simulink model "Copy_of_Esercizio8_sim"  (R2022a)
settings: Solver=VariableStepAuto  StartTime=0.0  StopTime=60  RelTol=1e-3
values from neighbouring files (symbols this model uses):
  PID_d = c2d (PID_continuo, Ts,'tustin')    [PID.m]
  Ts = 1/100    (= 0.01)    [PID.m]
undefined symbols (not defined in the file or in its folder): PI_discreto, PID_discreto
settings Model: Creator=chiar  LastModifiedBy=Stefano
settings SolverCC: AlgebraicLoopSolver=TrustRegion
settings DebuggingCC: UnconnectedInputMsg=warning  UnconnectedOutputMsg=warning  UnconnectedLineMsg=warning  SFMachineParentedDataDiag=warning
settings RTWCC: DLArmComputeVersion=19.05

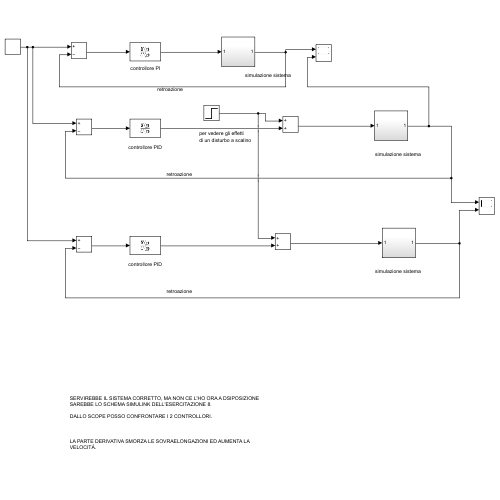
[thumbnail: Simulink's stored preview of the top-level diagram]
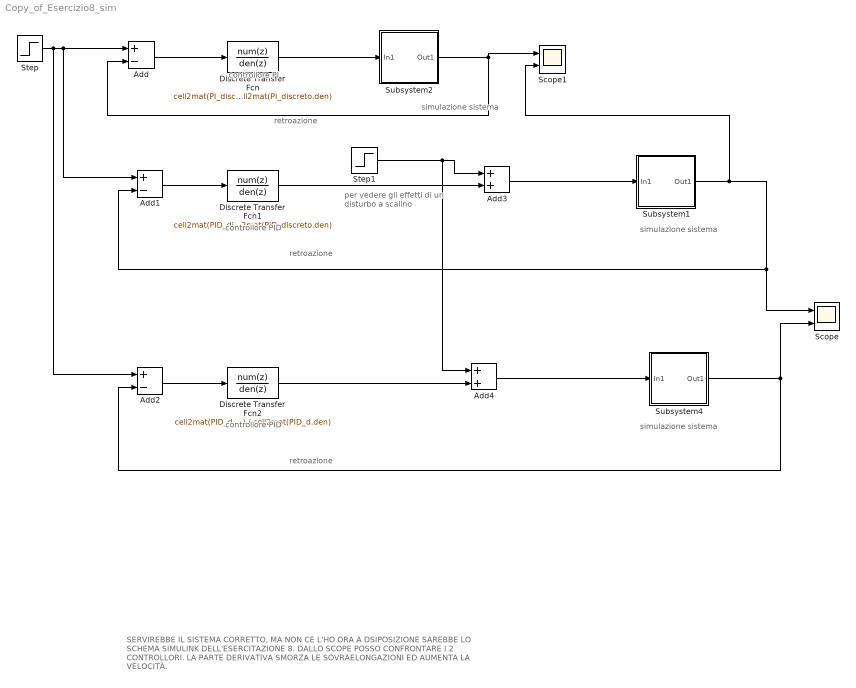
== system Copy_of_Esercizio8_sim ==
  note: per vedere gli effetti
      | di un disturbo a scalino
  note: SERVIREBBE IL SISTEMA CORRETTO, MA NON CE L'HO ORA A DSIPOSIZIONE
      | SAREBBE LO SCHEMA SIMULINK DELL'ESERCITAZIONE 8.
      |
      | DALLO SCOPE POSSO CONFRONTARE I 2 CONTROLLORI.
      |
      |
      |
      | LA PARTE DERIVATIVA SMORZA LE SOVRAELONGAZIONI ED AUMENTA LA VELOCITÀ.
  note: retroazione
  note: simulazione sistema
  note: controllore PID
  note: controllore PI
  note: simulazione sistema
  note: retroazione
  note: simulazione sistema
  note: controllore PID
  note: retroazione
  Add : Sum  Inputs=+-
  Add1 : Sum  Inputs=+-
  Add2 : Sum  Inputs=+-
  Add3 : Sum
  Add4 : Sum
  Discrete Transfer Fcn : DiscreteTransferFcn  Numerator=cell2mat(PI_discreto.num)  Denominator=cell2mat(PI_discreto.den)  SampleTime=Ts
  Discrete Transfer Fcn1 : DiscreteTransferFcn  Numerator=cell2mat(PID_discreto.num)  Denominator=cell2mat(PID_discreto.den)  SampleTime=Ts
  Discrete Transfer Fcn2 : DiscreteTransferFcn  Numerator=cell2mat(PID_d.num)  Denominator=cell2mat(PID_d.den)  SampleTime=Ts
  Scope : Scope  NumInputPorts=2
  Scope1 : Scope  NumInputPorts=2
  Step : Step  Time=0  SampleTime=0
  Step1 : Step  Time=30  After=0  SampleTime=0
  Subsystem1 : Subsystem
  Subsystem2 : Subsystem
  Subsystem4 : Subsystem
  wires:
  Discrete Transfer Fcn/1 -> Subsystem2/1(In1)
  Add1/1 -> Discrete Transfer Fcn1/1
  Add/1 -> Discrete Transfer Fcn/1
  Add2/1 -> Discrete Transfer Fcn2/1
  Subsystem4/1(Out1) -> Add2/2, Scope/2
  Step/1 -> Add2/1, Add1/1, Add/1
  Discrete Transfer Fcn1/1 -> Add3/2
  Add3/1 -> Subsystem1/1(In1)
  Step1/1 -> Add4/1, Add3/1
  Discrete Transfer Fcn2/1 -> Add4/2
  Subsystem1/1(Out1) -> Scope1/2, Scope/1, Add1/2
  Add4/1 -> Subsystem4/1(In1)
  Subsystem2/1(Out1) -> Add/2, Scope1/1

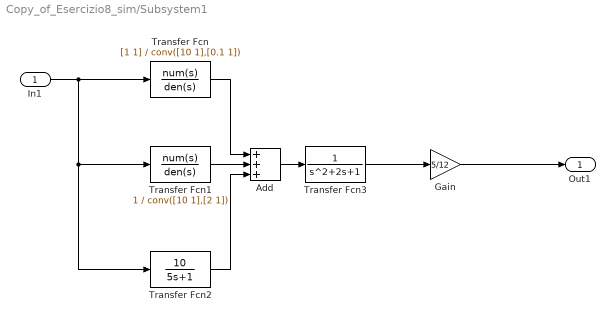
== system Copy_of_Esercizio8_sim/Subsystem1 ==
  In1 : Inport
  Add : Sum  Inputs=+++
  Gain : Gain  Gain=5/12
  Transfer Fcn : TransferFcn  Numerator=[1 1]  Denominator=conv([10 1],[0.1 1])
  Transfer Fcn1 : TransferFcn  Numerator=1  Denominator=conv([10 1],[2 1])
  Transfer Fcn2 : TransferFcn  Numerator=10  Denominator=[5 1]
  Transfer Fcn3 : TransferFcn  Numerator=1
  Out1 : Outport
  wires:
  Gain/1 -> Out1/1
  Transfer Fcn3/1 -> Gain/1
  Transfer Fcn2/1 -> Add/3
  Add/1 -> Transfer Fcn3/1
  Transfer Fcn/1 -> Add/1
  Transfer Fcn1/1 -> Add/2
  In1/1 -> Transfer Fcn/1, Transfer Fcn1/1, Transfer Fcn2/1

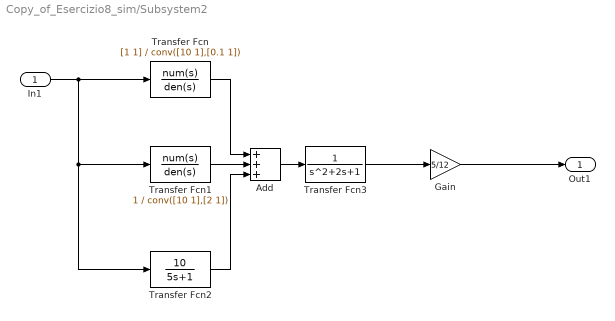
== system Copy_of_Esercizio8_sim/Subsystem2 ==
  In1 : Inport
  Add : Sum  Inputs=+++
  Gain : Gain  Gain=5/12
  Transfer Fcn : TransferFcn  Numerator=[1 1]  Denominator=conv([10 1],[0.1 1])
  Transfer Fcn1 : TransferFcn  Numerator=1  Denominator=conv([10 1],[2 1])
  Transfer Fcn2 : TransferFcn  Numerator=10  Denominator=[5 1]
  Transfer Fcn3 : TransferFcn  Numerator=1
  Out1 : Outport
  wires:
  Gain/1 -> Out1/1
  Transfer Fcn3/1 -> Gain/1
  Transfer Fcn2/1 -> Add/3
  Add/1 -> Transfer Fcn3/1
  Transfer Fcn/1 -> Add/1
  Transfer Fcn1/1 -> Add/2
  In1/1 -> Transfer Fcn/1, Transfer Fcn1/1, Transfer Fcn2/1

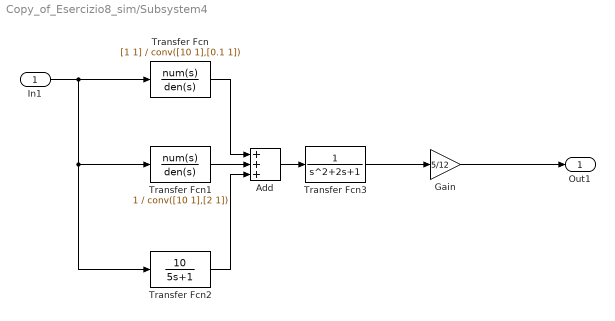
== system Copy_of_Esercizio8_sim/Subsystem4 ==
  In1 : Inport
  Add : Sum  Inputs=+++
  Gain : Gain  Gain=5/12
  Transfer Fcn : TransferFcn  Numerator=[1 1]  Denominator=conv([10 1],[0.1 1])
  Transfer Fcn1 : TransferFcn  Numerator=1  Denominator=conv([10 1],[2 1])
  Transfer Fcn2 : TransferFcn  Numerator=10  Denominator=[5 1]
  Transfer Fcn3 : TransferFcn  Numerator=1
  Out1 : Outport
  wires:
  Gain/1 -> Out1/1
  Transfer Fcn3/1 -> Gain/1
  Transfer Fcn2/1 -> Add/3
  Add/1 -> Transfer Fcn3/1
  Transfer Fcn/1 -> Add/1
  Transfer Fcn1/1 -> Add/2
  In1/1 -> Transfer Fcn/1, Transfer Fcn1/1, Transfer Fcn2/1
